simulink model "BD_PAR_AUTO_base_model"  (Simulink 10.3)
settings: Solver=ode1  StartTime=0.0  StopTime=max(cyc_mph(:,1))  FixedStep=1  MaxStep=1  RelTol=1e-3  AbsTol=1e-3
undefined symbols (not defined in the file): acc_dcdc_eff, acc_elec_eff, acc_elec_pwr, acc_mech_eff, acc_mech_pwr, acc_mech_trq, air_cp, amb_tmp, cs_charge_deplete_bool, cs_charge_trq, cs_electric_decel_spd, cs_electric_launch_spd_hi, cs_electric_launch_spd_lo, cs_hi_soc, cs_lo_soc, cs_min_trq_frac, cs_off_trq_frac, cyc_avg_time, cyc_cargo_mass, cyc_elevation_init, cyc_filter_bool, cyc_grade, cyc_mph, enable_sim_stop_distance, enable_sim_stop_max_spd, enable_sim_stop_speed, enable_sim_stop_time, enable_stop, enable_stop_fc, ess_cap_scale, ess_coulombic_eff, ess_init_soc, ess_max_ah_cap, ess_max_volts, ess_min_volts, ess_mod_airflow, ess_mod_cp, ess_mod_init_tmp, ess_module_mass, ess_module_num, ess_on, ess_r_chg, ess_r_dis, ess_res_scale_coef, ess_res_scale_fun, ess_set_tmp, ess_soc, ess_th_calc, ess_th_res_off, ess_th_res_on, ess_tmp, ess_voc, ex_calc, ex_cat_co_frac, ex_cat_ext_cp, ex_cat_ext_emisv, ex_cat_ext_init_tmp, ex_cat_ext_mass, ex_cat_ext_sarea, ex_cat_hc_frac ... (+168)
(part 6 of 15)

== system BD_PAR_AUTO_base_model/motor/ controller <mc> par/N-m drive torque per W input/Block NOTES ==
  note: This block determines the ratio of req'd rotor torque to req'd electrical input power,
      |  which is proportional to efficiency if the motor is providing torque.  This ratio is used
      | to compute actual rotor torque given some input power which may be different from
      | the req'd value.
      |
      | If the denominator, the req'd input power, is zero, this block outputs inf,
      | which is a flag used by the block .../rotor drive torque available (Nm).

== system BD_PAR_AUTO_base_model/motor/ controller <mc> par/effect of inertia (Nm)/Block NOTES ==
  note: Torque required to accelerate the motor's inertia is calculated from the rate of change
      | of mc_spd_out_a.  It is no greater than the product of the maximum motor torque and
      | the fractional contribution of the motor's inertia to the total vehicle inertia.

== system BD_PAR_AUTO_base_model/motor/ controller <mc> par/effect of inertia (Nm)/motor inertia as a function of total vehicle inertia (generous approximation) ==
  gear ratio : Inport
  Product : Product  Inputs=*/  SaturateOnIntegerOverflow=on
  Sum : Sum  Inputs=++|  SaturateOnIntegerOverflow=on
  engine inertia as a fraction of total vehicle inertia  (generous approximation)--denomenator : Fcn  Expr=mc_inertia*u^2
  engine inertia as a fraction of total vehicle inertia  (generous approximation)--numerator : Fcn  Expr=mc_inertia*u^2
  veh mass calc : Subsystem
  Out1 : Outport
  wires:
  Sum/1 -> Product/2
  engine inertia as a fraction of total vehicle inertia  (generous approximation)--denomenator/1 -> Sum/2
  veh mass calc/1(Out1) -> Sum/1
  gear ratio/1 -> engine inertia as a fraction of total vehicle inertia  (generous approximation)--denomenator/1, engine inertia as a fraction of total vehicle inertia  (generous approximation)--numerator/1
  Product/1 -> Out1/1
  engine inertia as a fraction of total vehicle inertia  (generous approximation)--numerator/1 -> Product/1

== system BD_PAR_AUTO_base_model/motor/ controller <mc> par/enforce torque limit/Block NOTES ==
  note: This block enforces the maximum torque production and absorption
      | capability limits of the motor.  It assumes that exactly as much torque
      | can be absorbed as can be produced at a given speed.

== system BD_PAR_AUTO_base_model/motor/ controller <mc> par/mc tmp/Block NOTES ==
  note: This block models the thermal behavior of a motor
      | and controller  with active fluid cooling.
      | The module is modeled as a single lumped thermal mass.
      | The fan is on whenever the battery temp is > the set temp.

== system BD_PAR_AUTO_base_model/motor/ controller <mc> par/mc tmp/mc coolant ==
  Tcl : Inport
  "Qmc " : Inport  Port=2
  Enable : EnablePort  StatesWhenEnabling=reset
  Constant : Constant  Value=mc_tstat
  Product1 : Product  SaturateOnIntegerOverflow=on
  Relational Operator : RelationalOperator  Operator=<=  RndMeth=Nearest  InputSameDT=on
  Qmc_clt : Outport  OutputWhenDisabled=reset  InitialOutput=0
  wires:
  Tcl/1 -> Relational Operator/2
  Constant/1 -> Relational Operator/1
  "Qmc "/1 -> Product1/2
  Product1/1 -> Qmc_clt/1
  Relational Operator/1 -> Product1/1

== system BD_PAR_AUTO_base_model/motor/ controller <mc> par/motor speed estimator/Block NOTES ==
  note: The requested motor speed is replaced by an estimate of the
      | motor's previous speed, for loss and max. torque calculations,
      | whenever the vehicle missed the trace by more than 1 mph
      | on the last time step.

== system BD_PAR_AUTO_base_model/motor/ controller <mc> par/rotor drive torque available (Nm)/Block NOTES ==
  note: This block computes the actual rotor torque given the actual motor input power and
      | the ratio (req'd rotor torque)/(req'd input power).
      |
      | If the above ratio has the value inf, which implies that the req'd input power is zero,
      | then the actual rotor torque is assumed to be zero.  This is not reflective of reality, of course:
      | with zero input power, the rotor torque would be the motor spin-loss torque at the given speed.
      | Because this simplification occurs only when req'd input power is zero, it does not.
      | affect fuel economy or max effort acceleration calculations.

== system BD_PAR_AUTO_base_model/vehicle <veh>/force req'd to accelerate (N)/current veh mass ==
  Constant3 : Constant  Value=veh_mass
  Sum1 : Sum  Inputs=|++  SaturateOnIntegerOverflow=on
  Out1 : Outport
  wires:
  Constant3/1 -> Sum1/1
  [veh_cargo_mass] -> Sum1/2
  Sum1/1 -> Out1/1

== system BD_PAR_AUTO_base_model/vehicle <veh>/force req'd to ascend (N)/current veh mass ==
  Constant3 : Constant  Value=veh_mass
  Sum1 : Sum  Inputs=|++  SaturateOnIntegerOverflow=on
  Out1 : Outport
  wires:
  Constant3/1 -> Sum1/1
  [veh_cargo_mass] -> Sum1/2
  Sum1/1 -> Out1/1

== system BD_PAR_AUTO_base_model/vehicle <veh>/record achieved force outputs/force req'd to accelerate (N)1 ==
  v(m/s) : Inport
  v prev : Inport  Port=2
  Clock : Clock
  Memory : Memory  InitialCondition=-0.1
  Product1 : Product  Inputs=**/  SaturateOnIntegerOverflow=on
  Sum : Sum  Inputs=+-  SaturateOnIntegerOverflow=on
  Sum1 : Sum  Inputs=+-  SaturateOnIntegerOverflow=on
  current veh mass : Subsystem
  (N) : Outport  InitialOutput=0
  wires:
  current veh mass/1(Out1) -> Product1/1
  Clock/1 -> Sum1/1, Memory/1
  Memory/1 -> Sum1/2
  Product1/1 -> (N)/1
  v prev/1 -> Sum/2
  v(m/s)/1 -> Sum/1
  Sum1/1 -> Product1/3
  Sum/1 -> Product1/2

== system BD_PAR_AUTO_base_model/vehicle <veh>/record achieved force outputs/force req'd to ascend (N)1 ==
  average vehicle speed over time step (m/s) : Inport
  Constant : Constant  Value=veh_gravity
  Constant1 : Constant  Value=0
  Product : Product  Inputs=3  SaturateOnIntegerOverflow=on
  Switch : Switch
  Trigonometric Function : Trigonometry  Operator=atan
  Trigonometric Function1 : Trigonometry
  current veh mass : Subsystem
  (N) : Outport  InitialOutput=0
  wires:
  current veh mass/1(Out1) -> Product/3
  average vehicle speed over time step (m/s)/1 -> Switch/2
  Constant1/1 -> Switch/3
  Switch/1 -> (N)/1
  Product/1 -> Switch/1
  Constant/1 -> Product/1
  [grade] -> Trigonometric Function/1
  Trigonometric Function1/1 -> Product/2
  Trigonometric Function/1 -> Trigonometric Function1/1

== system BD_PAR_AUTO_base_model/vehicle <veh>/record achieved force outputs/force req'd to overcome aerodynamic drag (N)1 ==
  average vehicle speed over time step (m/s) : Inport
  Constant : Constant  Value=veh_air_density*veh_CD*veh_FA*0.5
  Product : Product  Inputs=3  SaturateOnIntegerOverflow=on
  D aero(N) : Outport  InitialOutput=0
  wires:
  Product/1 -> D aero(N)/1
  Constant/1 -> Product/3
  average vehicle speed over time step (m/s)/1 -> Product/2, Product/1

== system BD_PAR_AUTO_base_model/vehicle <veh>/record achieved force outputs/rolling resistance force ==
  average vehicle speed over time step (m/s) : Inport
  force req'd to overcome rolling resistance (N) : Subsystem
  Fr (N) : Outport
  wires:
  average vehicle speed over time step (m/s)/1 -> force req'd to overcome rolling resistance (N)/1(average vehicle speed over time step (m/s))
  force req'd to overcome rolling resistance (N)/1(Fr (N)) -> Fr (N)/1

== system BD_PAR_AUTO_base_model/vehicle <veh>/rolling resistance force/force req'd to overcome rolling resistance (N) ==
  average vehicle speed over time step (m/s) : Inport
  Constant : Constant  Value=wh_1st_rrc
  Constant1 : Constant  Value=0
  Constant2 : Constant  Value=veh_gravity
  Gain1 : Gain  Gain=wh_2nd_rrc  SaturateOnIntegerOverflow=on
  Product : Product  Inputs=4  SaturateOnIntegerOverflow=on
  Sum : Sum  SaturateOnIntegerOverflow=on
  Switch : Switch  Threshold=eps
  Trig Fn2 : Trigonometry  Operator=atan
  Trig Fn3 : Trigonometry  Operator=cos
  current veh mass : Subsystem
  Fr (N) : Outport  InitialOutput=0
  wires:
  Constant/1 -> Sum/1
  Gain1/1 -> Sum/2
  Switch/1 -> Fr (N)/1
  average vehicle speed over time step (m/s)/1 -> Gain1/1, Switch/2
  Constant1/1 -> Switch/3
  Sum/1 -> Product/2
  Constant2/1 -> Product/1
  Product/1 -> Switch/1
  Trig Fn3/1 -> Product/3
  current veh mass/1(Out1) -> Product/4
  [grade] -> Trig Fn2/1
  Trig Fn2/1 -> Trig Fn3/1

== system BD_PAR_AUTO_base_model/vehicle <veh>/vehicle speed/vehicle speed (m/s) ==
  vehicle speed at beginning of time step (m/s) : Inport
  "available tractive force and linear speed (N), (m/s)" : Inport  Port=2
  Block NOTES : Subsystem
      mask Display: disp('Block\nNOTES')
  Clock : Clock
  Constant : Constant  Value=0
  Demux : Demux  Outputs=2
  Gain : Gain  Gain=-1  SaturateOnIntegerOverflow=on
  Gain1 : Gain  Gain=2  SaturateOnIntegerOverflow=on
  Memory : Memory  InitialCondition=-.1
  MinMax : MinMax  Inputs=2
  MinMax1 : MinMax  Function=max  Inputs=2
  Mux : Mux  Inputs=3
  Relational Operator : RelationalOperator  RndMeth=Nearest  InputSameDT=on
  Sum5 : Sum  Inputs=-+  SaturateOnIntegerOverflow=on
  Switch : Switch  Threshold=0.5
  Switch1 : Switch  Threshold=1e-9
  Trig Fn4 : Trigonometry  Operator=atan
  a : Constant  Value=0.5*veh_air_density*veh_CD*veh_FA
  b : Subsystem
  c : Subsystem
  current veh mass : Subsystem
  dt : Sum  Inputs=+-  SaturateOnIntegerOverflow=on
  only have rolling resistance if moving : Fcn  Expr=u>0
  solve the quadratic for avg. linear spd : Fcn  Expr=(-u[2]+(u[2]^2-4*u[1]*u[3])^.5)/(2*u[1])
  vehicle speed achievable at end of time step (m/s) : Outport  InitialOutput=0
  wires:
  vehicle speed at beginning of time step (m/s)/1 -> Sum5/1, c/2(v_prev)
  Demux/1 -> c/3(Ftract), Relational Operator/1
  Demux/2 -> MinMax1/2, MinMax/2, only have rolling resistance if moving/1
  c/1(c) -> Mux/3
  "available tractive force and linear speed (N), (m/s)"/1 -> Demux/1
  Constant/1 -> Switch1/3
  Sum5/1 -> Switch1/2, Switch1/1
  only have rolling resistance if moving/1 -> c/5(vehicle moving?), b/3(vehicle moving?)
  Trig Fn4/1 -> c/4(angle of elevation), b/2(angle of elevation)
  dt/1 -> c/1(dt), b/1(dt)
  [grade] -> Trig Fn4/1
  Memory/1 -> dt/2
  Clock/1 -> Memory/1, dt/1
  b/1(b) -> Mux/2
  Switch1/1 -> vehicle speed achievable at end of time step (m/s)/1
  Mux/1 -> solve the quadratic for avg. linear spd/1
  a/1 -> Mux/1
  MinMax/1 -> Switch/1
  MinMax1/1 -> Switch/3
  Gain1/1 -> Sum5/2
  solve the quadratic for avg. linear spd/1 -> MinMax1/1, MinMax/1
  Switch/1 -> Gain1/1
  Gain/1 -> Relational Operator/2
  current veh mass/1(Out1) -> Gain/1
  Relational Operator/1 -> Switch/2

== system BD_PAR_AUTO_base_model/wheel and axle  front/rear <wh>/front force/brake request  controller interface ==
  F_front_brake_req : Outport  InitialOutput=0
  wires:
  [F_front_brake_req] -> F_front_brake_req/1

== system BD_PAR_AUTO_base_model/wheel and axle  front/rear <wh>/loss (Nm)/veh mass calc ==
  Constant : Constant  Value=veh_mass
  Sum : Sum  Inputs=|++  SaturateOnIntegerOverflow=on
  Out1 : Outport
  wires:
  Sum/1 -> Out1/1
  Constant/1 -> Sum/2
  [veh_cargo_mass] -> Sum/1

== system BD_PAR_AUTO_base_model/wheel and axle  front/rear <wh>/rear force/brake request controller interface1 ==
  F_rear_brake_req : Outport  InitialOutput=0
  wires:
  [F_rear_brake_req] -> F_rear_brake_req/1

== system BD_PAR_AUTO_base_model/wheel and axle  front/rear <wh>/tire slip model (m/s)/Block NOTES ==
  note: This block implements the effects of finite tire slip (with respect to the road) on the
      | vehicle speed/wheel speed relationship.  Slip is defined as s=(omega*r - v) / v.  The
      | one-to-one mapping of slip to normalized tractive force, F_tract/W_front_axle, up to
      | the maximum, is stored in the variables "wh_slip" and "wh_slip_force_coeff."  The
      | slip calculation here is overridden if the actual axle speed and the requested axle
      | speed are the same, indicating that no drivetrain speed limits were encountered.

== system BD_PAR_AUTO_base_model/wheel and axle  front/rear <wh>/tire slip model (m/s)/front axle ==
  In1 : Inport
  In2 : Inport  Port=2
  Abs : Abs
  Constant3 : Constant  Value=0
  F/W : Product  Inputs=*/  SaturateOnIntegerOverflow=on
  Product : Product  SaturateOnIntegerOverflow=on
  Relational Operator : RelationalOperator  Operator=~=  RndMeth=Nearest  InputSameDT=on
  Saturation : Saturate  UpperLimit=max(wh_slip_force_coeff)  LowerLimit=min(wh_slip_force_coeff)
  Sign : Signum
  Switch : Switch
  s=s(F/W) : Lookup  InputValues=wh_slip_force_coeff  Table=wh_slip
  Out1 : Outport
  wires:
  Product/1 -> Out1/1
  In1/1 -> F/W/2
  In2/1 -> Sign/1, Abs/1
  s=s(F/W)/1 -> Product/1
  Sign/1 -> Product/2
  F/W/1 -> Switch/1
  Switch/1 -> Saturation/1
  Saturation/1 -> s=s(F/W)/1
  Abs/1 -> Relational Operator/1, F/W/1
  Relational Operator/1 -> Switch/2
  Constant3/1 -> Relational Operator/2, Switch/3

== system BD_PAR_AUTO_base_model/wheel and axle  front/rear <wh>/tire slip model (m/s)/rear axle ==
  In1 : Inport
  In2 : Inport  Port=2
  Abs : Abs
  Constant3 : Constant  Value=0
  F/W : Product  Inputs=*/  SaturateOnIntegerOverflow=on
  Product : Product  SaturateOnIntegerOverflow=on
  Relational Operator : RelationalOperator  Operator=~=  RndMeth=Nearest  InputSameDT=on
  Saturation : Saturate  UpperLimit=max(wh_slip_force_coeff)  LowerLimit=min(wh_slip_force_coeff)
  Sign : Signum
  Switch : Switch
  s=s(F/W) : Lookup  InputValues=wh_slip_force_coeff  Table=wh_slip
  Out1 : Outport
  wires:
  Product/1 -> Out1/1
  In1/1 -> F/W/2
  In2/1 -> Sign/1, Abs/1
  s=s(F/W)/1 -> Product/1
  Sign/1 -> Product/2
  F/W/1 -> Switch/1
  Switch/1 -> Saturation/1
  Saturation/1 -> s=s(F/W)/1
  Abs/1 -> Relational Operator/1, F/W/1
  Relational Operator/1 -> Switch/2
  Constant3/1 -> Relational Operator/2, Switch/3

== system BD_PAR_AUTO_base_model/wheel and axle  front/rear <wh>/tire slip model (rad/s)/front slip ==
  In1 : Inport
  In2 : Inport  Port=2
  Abs : Abs
  F/W : Product  Inputs=*/  SaturateOnIntegerOverflow=on
  Product : Product  SaturateOnIntegerOverflow=on
  Saturation : Saturate  UpperLimit=max(wh_slip_force_coeff)  LowerLimit=min(wh_slip_force_coeff)
  Sign : Signum
  s=s(F/W) : Lookup  InputValues=wh_slip_force_coeff  Table=wh_slip
  Out1 : Outport
  wires:
  Product/1 -> Out1/1
  In1/1 -> F/W/2
  s=s(F/W)/1 -> Product/1
  In2/1 -> Sign/1, Abs/1
  Sign/1 -> Product/2
  Abs/1 -> F/W/1
  F/W/1 -> Saturation/1
  Saturation/1 -> s=s(F/W)/1

== system BD_PAR_AUTO_base_model/wheel and axle  front/rear <wh>/tire slip model (rad/s)/rear slip ==
  In1 : Inport
  In2 : Inport  Port=2
  Abs : Abs
  F/W : Product  Inputs=*/  SaturateOnIntegerOverflow=on
  Product : Product  SaturateOnIntegerOverflow=on
  Saturation : Saturate  UpperLimit=max(wh_slip_force_coeff)  LowerLimit=min(wh_slip_force_coeff)
  Sign : Signum
  s=s(F/W) : Lookup  InputValues=wh_slip_force_coeff  Table=wh_slip
  Out1 : Outport
  wires:
  Product/1 -> Out1/1
  In1/1 -> F/W/2
  s=s(F/W)/1 -> Product/1
  In2/1 -> Sign/1, Abs/1
  Sign/1 -> Product/2
  Abs/1 -> F/W/1
  F/W/1 -> Saturation/1
  Saturation/1 -> s=s(F/W)/1

== system BD_PAR_AUTO_base_model/<vc> par auto/config traction control/traction control 2 axle/Block NOTES ==
  note: Requested speed and force are limited by the
      | tractive characteristics of the tires in this block.

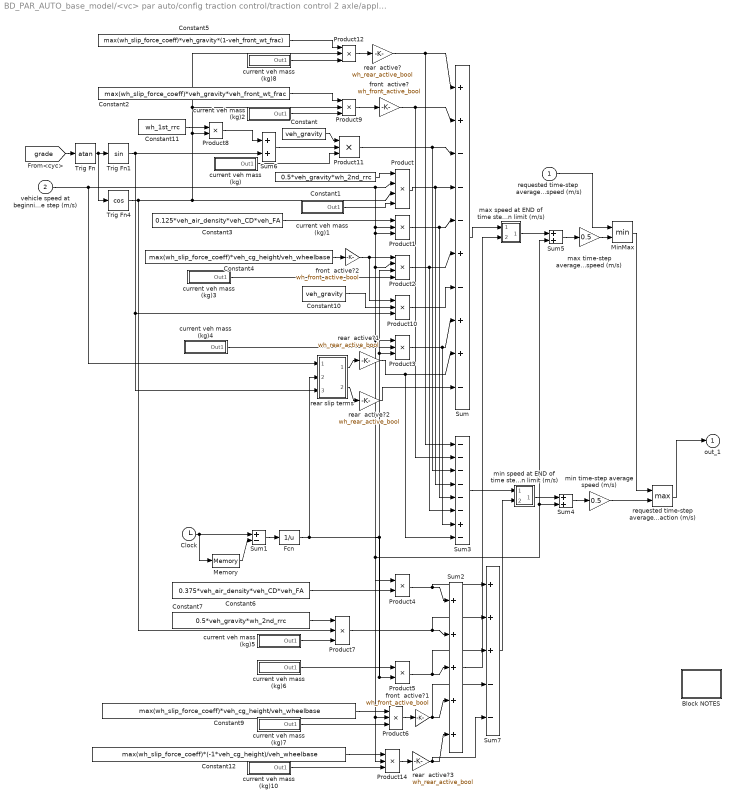
== system BD_PAR_AUTO_base_model/<vc> par auto/config traction control/traction control 2 axle/apply tire traction limit to req'd speed (m/s) ==
  "requested time-step  average vehicle speed (m/s) " : Inport
  vehicle speed at beginning of time step (m/s) : Inport  Port=2
  Block NOTES : Subsystem
      mask Display: disp('Block\nNOTES')
  Clock : Clock
  Constant : Constant  Value=veh_gravity
  Constant1 : Constant  Value=0.5*veh_gravity*wh_2nd_rrc
  Constant10 : Constant  Value=veh_gravity
  Constant11 : Constant  Value=wh_1st_rrc
  Constant12 : Constant  Value=max(wh_slip_force_coeff)*(-1*veh_cg_height)/veh_wheelbase
  Constant2 : Constant  Value=max(wh_slip_force_coeff)*veh_gravity*veh_front_wt_frac
  Constant3 : Constant  Value=0.125*veh_air_density*veh_CD*veh_FA
  Constant4 : Constant  Value=max(wh_slip_force_coeff)*veh_cg_height/veh_wheelbase
  Constant5 : Constant  Value=max(wh_slip_force_coeff)*veh_gravity*(1-veh_front_wt_frac)
  Constant6 : Constant  Value=0.375*veh_air_density*veh_CD*veh_FA
  Constant7 : Constant  Value=0.5*veh_gravity*wh_2nd_rrc
  Constant9 : Constant  Value=max(wh_slip_force_coeff)*veh_cg_height/veh_wheelbase
  Fcn : Fcn  Expr=1/u
  Memory : Memory  InitialCondition=-0.1
  MinMax : MinMax  Inputs=2  InputSameDT=on  SaturateOnIntegerOverflow=on
  Product : Product  Inputs=4  InputSameDT=on  RndMeth=Zero  SaturateOnIntegerOverflow=on  OutDataTypeStr=Inherit: Same as first input
  Product{1,3,6..7,9..12,14} (9 alike) : Product  Inputs=3  InputSameDT=on  RndMeth=Zero  SaturateOnIntegerOverflow=on  OutDataTypeStr=Inherit: Same as first input
  Product2 : Product  Inputs=4  InputSameDT=on  RndMeth=Zero  SaturateOnIntegerOverflow=on  OutDataTypeStr=Inherit: Same as first input
  Product4 : Product  InputSameDT=on  RndMeth=Zero  SaturateOnIntegerOverflow=on  OutDataTypeStr=Inherit: Same as first input
  Product5 : Product  InputSameDT=on  RndMeth=Zero  SaturateOnIntegerOverflow=on  OutDataTypeStr=Inherit: Same as first input
  Product8 : Product  InputSameDT=on  RndMeth=Zero  SaturateOnIntegerOverflow=on  OutDataTypeStr=Inherit: Same as first input
  Sum : Sum  Inputs=++---+-++-  InputSameDT=on  SaturateOnIntegerOverflow=on  OutDataTypeStr=Inherit: Same as first input
  Sum1 : Sum  Inputs=+-  InputSameDT=on  SaturateOnIntegerOverflow=on  OutDataTypeStr=Inherit: Same as first input
  Sum2 : Sum  Inputs=+++++  InputSameDT=on  SaturateOnIntegerOverflow=on  OutDataTypeStr=Inherit: Same as first input
  Sum3 : Sum  Inputs=------+-  InputSameDT=on  SaturateOnIntegerOverflow=on  OutDataTypeStr=Inherit: Same as first input
  Sum4 : Sum  InputSameDT=on  SaturateOnIntegerOverflow=on  OutDataTypeStr=Inherit: Same as first input
  Sum5 : Sum  InputSameDT=on  SaturateOnIntegerOverflow=on  OutDataTypeStr=Inherit: Same as first input
  Sum6 : Sum  InputSameDT=on  SaturateOnIntegerOverflow=on  OutDataTypeStr=Inherit: Same as first input
  Sum7 : Sum  Inputs=+++--  InputSameDT=on  SaturateOnIntegerOverflow=on  OutDataTypeStr=Inherit: Same as first input
  Trig Fn4 : Trigonometry  Operator=cos
  Trig Fn : Trigonometry  Operator=atan
  Trig Fn1 : Trigonometry
  current veh mass (kg) : Subsystem
  current veh mass (kg)1 : Subsystem
  current veh mass (kg)10 : Subsystem
  current veh mass (kg)2 : Subsystem
  current veh mass (kg)3 : Subsystem
  current veh mass (kg)4 : Subsystem
  current veh mass (kg)5 : Subsystem
  current veh mass (kg)6 : Subsystem
  current veh mass (kg)7 : Subsystem
  current veh mass (kg)8 : Subsystem
  front  active? : Gain  Gain=wh_front_active_bool  SaturateOnIntegerOverflow=on  OutDataTypeStr=Inherit: Same as input  ParamDataTypeStr=Inherit: Same as input
  front  active?1 : Gain  Gain=wh_front_active_bool  SaturateOnIntegerOverflow=on  OutDataTypeStr=Inherit: Same as input  ParamDataTypeStr=Inherit: Same as input
  front  active?2 : Gain  Gain=wh_front_active_bool  SaturateOnIntegerOverflow=on  OutDataTypeStr=Inherit: Same as input  ParamDataTypeStr=Inherit: Same as input
  max speed at END of time step given tire traction limit (m/s) : Subsystem
      mask Display: disp('/')
  max time-step average speed (m/s) : Gain  Gain=0.5  SaturateOnIntegerOverflow=on  OutDataTypeStr=Inherit: Same as input  ParamDataTypeStr=Inherit: Same as input
  min speed at END of time step given tire traction limit (m/s) : Subsystem
      mask Display: disp('/')
  min time-step average speed (m/s) : Gain  Gain=0.5  SaturateOnIntegerOverflow=on  OutDataTypeStr=Inherit: Same as input  ParamDataTypeStr=Inherit: Same as input
  rear  active?{,1..3} (4 alike) : Gain  Gain=wh_rear_active_bool  SaturateOnIntegerOverflow=on  OutDataTypeStr=Inherit: Same as input  ParamDataTypeStr=Inherit: Same as input
  rear slip terms : Subsystem
  requested time-step average speed limited by tire traction (m/s) : MinMax  Function=max  Inputs=2  InputSameDT=on  SaturateOnIntegerOverflow=on
  out_1 : Outport  InitialOutput=0
  wires:
  front  active?2/1 -> Product10/1, Product2/1
  front  active?1/1 -> Sum2/4, Sum7/4
  front  active?/1 -> Sum3/2, Sum/2
  rear  active?3/1 -> Sum2/5, Sum7/5
  rear  active?2/1 -> Sum/10
  rear  active?1/1 -> Sum3/8, Sum/9
  current veh mass (kg)10/1(Out1) -> Product14/3
  Constant12/1 -> Product14/1
  Product14/1 -> rear  active?3/1
  rear slip terms/2(Out2) -> rear  active?2/1
  rear slip terms/1(Out1) -> rear  active?1/1
  rear  active?/1 -> Sum3/1, Sum/1
  current veh mass (kg)8/1(Out1) -> Product12/3
  Constant5/1 -> Product12/1
  Product12/1 -> rear  active?/1
  current veh mass (kg)7/1(Out1) -> Product6/3
  current veh mass (kg)5/1(Out1) -> Product7/3
  current veh mass (kg)3/1(Out1) -> Product2/4
  current veh mass (kg)2/1(Out1) -> Product9/3
  current veh mass (kg)1/1(Out1) -> Product/4
  current veh mass (kg)/1(Out1) -> Product11/3
  Constant/1 -> Product11/1
  Product11/1 -> Sum3/3, Sum/3
  Sum6/1 -> Product11/2
  Trig Fn1/1 -> rear slip terms/3(sin(theta)), Product10/3, Sum6/2
  Constant10/1 -> Product10/2
  Constant4/1 -> front  active?2/1
  Product10/1 -> Sum/7
  Product3/1 -> Sum3/7, Sum/8
  current veh mass (kg)4/1(Out1) -> Product3/2
  max time-step average speed (m/s)/1 -> MinMax/2
  "requested time-step  average vehicle speed (m/s) "/1 -> MinMax/1
  Sum5/1 -> max time-step average speed (m/s)/1
  Constant2/1 -> Product9/1
  Constant11/1 -> Product8/1
  Product8/1 -> Sum6/1
  Trig Fn4/1 -> Product12/2, Product9/2, Product8/2, Product/3, Product7/2
  Clock/1 -> Memory/1, Sum1/1
  Sum1/1 -> Fcn/1
  Memory/1 -> Sum1/2
  current veh mass (kg)6/1(Out1) -> Product5/1
  Sum2/1 -> max speed at END of time step given tire traction limit (m/s)/2(in_2)
  min time-step average speed (m/s)/1 -> requested time-step average speed limited by tire traction (m/s)/2
  requested time-step average speed limited by tire traction (m/s)/1 -> out_1/1
  Sum4/1 -> min time-step average speed (m/s)/1
  min speed at END of time step given tire traction limit (m/s)/1(out_1) -> Sum4/1
  MinMax/1 -> requested time-step average speed limited by tire traction (m/s)/1
  Sum3/1 -> min speed at END of time step given tire traction limit (m/s)/1(in_1)
  Sum7/1 -> min speed at END of time step given tire traction limit (m/s)/2(in_2)
  Constant7/1 -> Product7/1
  Constant9/1 -> Product6/1
  Constant6/1 -> Product4/2
  Product4/1 -> Sum2/1, Sum7/1
  Product7/1 -> Sum2/2, Sum7/2
  Product5/1 -> Sum2/3, Sum7/3
  Product6/1 -> front  active?1/1
  Trig Fn/1 -> Trig Fn4/1, Trig Fn1/1
  vehicle speed at beginning of time step (m/s)/1 -> rear slip terms/1(initial speed), Sum5/2, Sum4/2, Product4/1, Product3/1, Product2/2, Product1/3, Product1/2, Product/2
  [grade] -> Trig Fn/1
  max speed at END of time step given tire traction limit (m/s)/1(out_1) -> Sum5/1
  Product2/1 -> Sum3/6, Sum/6
  Product9/1 -> front  active?/1
  Product/1 -> Sum3/4, Sum/4
  Product1/1 -> Sum3/5, Sum/5
  Sum/1 -> max speed at END of time step given tire traction limit (m/s)/1(in_1)
  Fcn/1 -> rear slip terms/2(1/dt), Product14/2, Product6/2, Product5/2, Product3/3, Product2/3
  Constant3/1 -> Product1/1
  Constant1/1 -> Product/1

== system BD_PAR_AUTO_base_model/<vc> par auto/config traction control/traction control 2 axle/enforce max.  front axle tractive force  due to slip (N) ==
  tractive force req'd at tire/road interface (N) : Inport
  requested time-step average vehicle speed (m/s) : Inport  Port=2
  speed at beginning of time step (m/s) : Inport  Port=3
  " " : MinMax  Inputs=2  InputSameDT=on  SaturateOnIntegerOverflow=on
  Block NOTES : Subsystem
      mask Display: disp('Block\nNOTES')
  Constant2 : Constant  Value=max(wh_slip_force_coeff)
  Gain : Gain  Gain=-1  SaturateOnIntegerOverflow=on  OutDataTypeStr=Inherit: Same as input  ParamDataTypeStr=Inherit: Same as input
  Product1 : Product  InputSameDT=on  RndMeth=Zero  SaturateOnIntegerOverflow=on  OutDataTypeStr=Inherit: Same as first input
  Product2 : Product  InputSameDT=on  RndMeth=Zero  SaturateOnIntegerOverflow=on  OutDataTypeStr=Inherit: Same as first input
  Product3 : Product  Inputs=*/  InputSameDT=on  RndMeth=Zero  SaturateOnIntegerOverflow=on  OutDataTypeStr=Inherit: Same as first input
  Product4 : Product  Inputs=*/  InputSameDT=on  RndMeth=Zero  SaturateOnIntegerOverflow=on  OutDataTypeStr=Inherit: Same as first input
  Sum1 : Sum  InputSameDT=on  SaturateOnIntegerOverflow=on  OutDataTypeStr=Inherit: Same as first input
  Sum2 : Sum  InputSameDT=on  SaturateOnIntegerOverflow=on  OutDataTypeStr=Inherit: Same as first input
  front : Subsystem
  front  active? : Gain  Gain=wh_front_active_bool  SaturateOnIntegerOverflow=on  OutDataTypeStr=Inherit: Same as input  ParamDataTypeStr=Inherit: Same as input
  front traction ratio : ToWorkspace  VariableName=front_traction_ratio_orig
  rear : Subsystem
  rear  active? : Gain  Gain=wh_rear_active_bool  SaturateOnIntegerOverflow=on  OutDataTypeStr=Inherit: Same as input  ParamDataTypeStr=Inherit: Same as input
  tractive force request limited by slip-threshhold force (N)1 : MinMax  Function=max  Inputs=2  InputSameDT=on  SaturateOnIntegerOverflow=on
  slip-limited force (N) : Outport  InitialOutput=0
  weight on front axle (N) : Outport  Port=2  InitialOutput=0
  weight on rear axle (N) : Outport  Port=3  InitialOutput=0
  front/total traction ratio : Outport  Port=4  InitialOutput=0
  wires:
  Product4/1 -> front traction ratio/1
  Sum2/1 -> Product4/2
  rear  active?/1 -> Sum1/2
  front  active?/1 -> Product3/1, Sum1/1
  Product3/1 -> front/total traction ratio/1
  Product2/1 -> Product4/1, Sum2/1, front  active?/1
  Product1/1 -> Sum2/2, rear  active?/1
  Sum1/1 -> Product3/2, Gain/1, " "/1
  rear/1(Out1) -> Product1/1, weight on rear axle (N)/1
  tractive force request limited by slip-threshhold force (N)1/1 -> slip-limited force (N)/1
  " "/1 -> tractive force request limited by slip-threshhold force (N)1/1
  tractive force req'd at tire/road interface (N)/1 -> " "/2
  Constant2/1 -> Product1/2, Product2/2
  Gain/1 -> tractive force request limited by slip-threshhold force (N)1/2
  speed at beginning of time step (m/s)/1 -> rear/2(In2), front/2(In2)
  requested time-step average vehicle speed (m/s)/1 -> rear/1(In1), front/1(In1)
  front/1(Out1) -> weight on front axle (N)/1, Product2/1

== system BD_PAR_AUTO_base_model/<vc> par auto/front and rear brake controller (achievable)/braking force supplied by front friction brakes (N)/Block NOTES ==
  note: If additional braking force is required to meet the specified deceleration, input #1 will be negative.
      | The fraction of the additional req'd braking force made up by the front-axle friction brakes is given by:
  note: [front_axle_friction_brake_fraction(vehicle speed)]
      | ------------------------------------------------------------------------------
      | [front_axle_friction_brake_fraction(vehicle speed) + rear_axle_friction_brake_fraction(vehicle speed)]
  note: where the denominator can also be expressed as [1 - front_axle_drivetrain_brake_fraction(vehicle speed)].
  note: If all braking was intended to be done by the drivetrain, the front friction brakes will do 60% of the braking.
  note: The variable "wh_max_front_fric_brake_force_N" must be assigned a positive value.

== system BD_PAR_AUTO_base_model/<vc> par auto/gearbox control for use w/ AT/Speed Dependent Shifting/shifting ==
  gear number : Inport
  Constant : Constant  Value=gb_shift_delay-1e-6
  Relational Operator : RelationalOperator  Operator=<  RndMeth=Nearest  InputSameDT=on
  time since last shift : Subsystem
      mask Display: disp('time since\nlast shift')
  out_1 : Outport  InitialOutput=0
  wires:
  time since last shift/1(out_1) -> Relational Operator/1
  Constant/1 -> Relational Operator/2
  gear number/1 -> time since last shift/1(in_1)
  Relational Operator/1 -> out_1/1

== system BD_PAR_AUTO_base_model/<vc> par auto/gearbox control for use w/ AT/Speed Dependent Shifting/shifting1 ==
  gear number : Inport
  Constant : Constant  Value=gb_shift_delay-1e-6
  Relational Operator : RelationalOperator  Operator=<  RndMeth=Nearest  InputSameDT=on
  time since last shift : Subsystem
      mask Display: disp('time since\nlast shift')
  out_1 : Outport  InitialOutput=0
  wires:
  time since last shift/1(out_1) -> Relational Operator/1
  Constant/1 -> Relational Operator/2
  gear number/1 -> time since last shift/1(in_1)
  Relational Operator/1 -> out_1/1

== system BD_PAR_AUTO_base_model/<vc> par auto/gearbox control for use w/ AT/downshift  command/load fraction ==
  In1 : Inport
  S-Function : S-Function  FunctionName=sfun_gearbox  Parameters=load, spd  SFunctionDeploymentMode=off  EnableBusSupport=off
  Out1 : Outport  InitialOutput=0
  wires:
  In1/1 -> S-Function/1
  S-Function/1 -> Out1/1

== system BD_PAR_AUTO_base_model/<vc> par auto/gearbox control for use w/ AT/downshift  command1/load fraction ==
  In1 : Inport
  S-Function : S-Function  FunctionName=sfun_gearbox  Parameters=load, spd  SFunctionDeploymentMode=off  EnableBusSupport=off
  Out1 : Outport  InitialOutput=0
  wires:
  S-Function/1 -> Out1/1
  In1/1 -> S-Function/1

== system BD_PAR_AUTO_base_model/<vc> par auto/gearbox control for use w/ AT/est. engine trq and spd/Block NOTES ==
  note: Estimate engine torque and speed associated with the previous gear, assuming that
      | the gearbox efficiency is constant.

== system BD_PAR_AUTO_base_model/<vc> par auto/gearbox control for use w/ AT/est. engine trq and spd/K_adv ==
  "Req'd output trq and spd (Nm), (rad/s)" : Inport
  K_adv=wout/(Tout)^0.5 : Fcn  Expr=u[2]/u[1]^0.5
  Saturation : Saturate  UpperLimit=max(htc_k_adv)  LowerLimit=min(htc_k_adv)
  Saturation2 : Saturate  UpperLimit=inf  LowerLimit=eps
  K_adv : Outport
  wires:
  Saturation/1 -> K_adv/1
  K_adv=wout/(Tout)^0.5/1 -> Saturation/1
  Saturation2/1 -> K_adv=wout/(Tout)^0.5/1
  "Req'd output trq and spd (Nm), (rad/s)"/1 -> Saturation2/1

== system BD_PAR_AUTO_base_model/<vc> par auto/gearbox control for use w/ AT/est. engine trq and spd assuming lockup/Block NOTES ==
  note: Estimate engine torque and speed associated with the current gear, assuming that
      | the gearbox efficiency is constant.

== system BD_PAR_AUTO_base_model/<vc> par auto/gearbox control for use w/ AT/shifting1/time since last shift ==
  in_1 : Inport
  just shifted : Subsystem
      mask Display: disp('just\nshifted')
  timer : Subsystem
      mask Display: disp('timer')
  out_1 : Outport  InitialOutput=0
  wires:
  timer/1(time) -> out_1/1
  just shifted/1(out_1) -> timer/1(trigger)
  in_1/1 -> just shifted/1(in_1)

== system BD_PAR_AUTO_base_model/<vc> par auto/gearbox control for use w/ AT/upshift  command/load fraction ==
  In1 : Inport
  S-Function : S-Function  FunctionName=sfun_gearbox  Parameters=load, spd  SFunctionDeploymentMode=off  EnableBusSupport=off
  Out1 : Outport  InitialOutput=0
  wires:
  In1/1 -> S-Function/1
  S-Function/1 -> Out1/1

== system BD_PAR_AUTO_base_model/<vc> par auto/parallel clutch control/gearbox speed estimator/Block NOTES ==
  note: The requested engine speed is replaced by an estimate of the
      | engine's previous speed whenever the vehicle missed the trace
      |  by more than 1 mph on the last time step.

== system BD_PAR_AUTO_base_model/<vc> par auto/parallel clutch control/gearbox speed estimator/dt ==
  Clock : Clock
  Memory1 : Memory  InitialCondition=-1
  Sum4 : Sum  Inputs=+-  InputSameDT=on  SaturateOnIntegerOverflow=on  OutDataTypeStr=Inherit: Same as first input
  Out1 : Outport  InitialOutput=0
  wires:
  Sum4/1 -> Out1/1
  Memory1/1 -> Sum4/2
  Clock/1 -> Memory1/1, Sum4/1

== system BD_PAR_AUTO_base_model/<vc> par auto/sim stop subsystem/stop sim max spd/Block NOTES ==
  note: When enabled, stop the simulation when the current speed is greater
      | than zero and is less than or equal to the speed at gb_shift_delay*5+1
      | seconds ago (i.e. vehicle has reached a constant max speed). Only used
      | during acceleration test.

== system BD_PAR_AUTO_base_model/electric acc loads <acc>/Electrical Accessory Loads v2 <acc>/Accessory SDO/electrical power logging ==
  In1 : Inport
  Gain : Gain  Gain=acc_elec_eff  SaturateOnIntegerOverflow=on  OutDataTypeStr=Inherit: Same as input  ParamDataTypeStr=Inherit: Same as input
  To Workspace6 : ToWorkspace  VariableName=acc_elec_pwr_in_a  SampleTime=-1
  To Workspace8 : ToWorkspace  VariableName=acc_elec_pwr_out_a  SampleTime=-1
  wires:
  Gain/1 -> To Workspace8/1
  In1/1 -> Gain/1, To Workspace6/1

== system BD_PAR_AUTO_base_model/electric acc loads <acc>/Electrical Accessory Loads v2 <acc>/backward model/electrical accessories (W) ==
  Electrical Accessories: Time Variable : Subsystem
      mask Display: image(imread('bdi_acc_elec_cs.bmp'))
  P_elec_acc : Outport
  wires:
  Electrical Accessories: Time Variable/1(P_elec_acc) -> P_elec_acc/1

== system BD_PAR_AUTO_base_model/energy storage <ess>/ess config/energy storage <ess>/Block NOTES ==
  note: This block models the energy storage system as an SOC-dependent voltage
      | in series with an SOC- and current direction-dependent internal resistance.
      | SOC is computed assuming that A-h capacity is constant, but limited
      | such that a minimum voltage is never exceeded (replacing the
      | previous Peukert relationship which underpredicted battery capacity).
      |
      | Discharge power is limited here so as not to bring the bus (battery pack) voltage below
      | the minimum controller voltage or the minimum battery voltage and so as to allow
      | the solution of the quadratic eq'n for discharge current.
      |
      | Charge current is limited to ensure the voltage does not exceed a maximum
      | voltage
      |
      | Positive current is discharge current in the convention used here.
      | Power loss is computed as I*R+losses due to Coulombic (in)efficiency.
      |
      | Thermal modeling of the battery performance is modeled in the
      | OCV, Rint, and capacity.

== system BD_PAR_AUTO_base_model/energy storage <ess>/ess config/energy storage <ess>/SOC algorithm ==
  note: SOC=(Max Ah capacity-Ah used)/Max Ah capacity
  (A) : Inport
  tmp (C) : Inport  Port=2
  (sec->hrs) : Gain  Gain=1/3600  SaturateOnIntegerOverflow=on  OutDataTypeStr=Inherit: Same as input  ParamDataTypeStr=Inherit: Same as input
  0 <= SOC <= 1 : Saturate  UpperLimit=1  LowerLimit=0
  A-h remaining : Sum  Inputs=-+  InputSameDT=on  SaturateOnIntegerOverflow=on  OutDataTypeStr=Inherit: Same as first input
  Ah used : Integrator  InitialConditionSource=external  InitialCondition=(1-ess_init_soc)*ess_max_ah_cap
  Fcn : Fcn  Expr=1/u
  Fcn1 : Fcn  Expr=(1-ess_init_soc)*u
  SOC : Product  InputSameDT=on  RndMeth=Zero  SaturateOnIntegerOverflow=on  OutDataTypeStr=Inherit: Same as first input
  Switch : Switch
  adjusted A : Product  InputSameDT=on  RndMeth=Zero  SaturateOnIntegerOverflow=on  OutDataTypeStr=Inherit: Same as first input
  coul eff : Lookup  InputValues=ess_tmp  Table=ess_coulombic_eff
  max cap : Lookup  InputValues=ess_tmp  Table=ess_max_ah_cap*ess_cap_scale
  SOC1 : Outport  InitialOutput=0
  wires:
  (A)/1 -> Switch/2, Switch/1, adjusted A/1
  Switch/1 -> (sec->hrs)/1
  (sec->hrs)/1 -> Ah used/1
  Ah used/1 -> A-h remaining/1
  Fcn/1 -> SOC/2
  SOC/1 -> 0 <= SOC <= 1/1
  A-h remaining/1 -> SOC/1
  0 <= SOC <= 1/1 -> SOC1/1
  tmp (C)/1 -> max cap/1, coul eff/1
  coul eff/1 -> adjusted A/2
  adjusted A/1 -> Switch/3
  max cap/1 -> A-h remaining/2, Fcn/1, Fcn1/1
  Fcn1/1 -> Ah used/2

== system BD_PAR_AUTO_base_model/energy storage <ess>/ess config/energy storage <ess>/compute current ==
  Voc : Inport
  Rint : Inport  Port=2
  limited output power (W) : Inport  Port=3
  Ibty=(Voc-(Voc^2-4RPbty)^.5)        ----------------------------- (2*R) : Fcn  Expr=(u[2]-(u[2]^2-4*u[1]*u[3])^.5)/(2*u[3])
  Logical Operator1 : Logic  Operator=NOT  Inputs=1
  Mux3 : Mux  Inputs=3
  Mux4 : Mux  Inputs=3
  Mux5 : Mux  Inputs=3
  To Workspace9 : ToWorkspace  VariableName=ess_current  SampleTime=-1
  Voc-I*R : Fcn  Expr=u[2]-u[1]*u[3]
  ess max voltage*#batts : Constant  Value=ess_max_volts*ess_module_num
  iabs min=(Voc-Vmax)/R : Fcn  Expr=(u(1)-u(2))/u(3)
  limit current based on  max voltage during charge : Switch  Threshold=eps
  min charge current not exceeded : RelationalOperator  Operator=>  RndMeth=Nearest  InputSameDT=on
  I_ : Outport  InitialOutput=0
  V_ : Outport  Port=2  InitialOutput=0
  tag scope: ess_maxV_limited=global
  wires:
  limited output power (W)/1 -> Mux4/1
  Voc/1 -> Mux4/2, Mux3/2, Mux5/1
  Rint/1 -> Mux4/3, Mux3/3, Mux5/3
  Ibty=(Voc-(Voc^2-4RPbty)^.5)        ----------------------------- (2*R)/1 -> min charge current not exceeded/1, limit current based on  max voltage during charge/1
  iabs min=(Voc-Vmax)/R/1 -> min charge current not exceeded/2, limit current based on  max voltage during charge/3
  limit current based on  max voltage during charge/1 -> I_/1, To Workspace9/1, Mux3/1
  min charge current not exceeded/1 -> limit current based on  max voltage during charge/2, Logical Operator1/1
  Mux3/1 -> Voc-I*R/1
  Voc-I*R/1 -> V_/1
  Mux4/1 -> Ibty=(Voc-(Voc^2-4RPbty)^.5)        ----------------------------- (2*R)/1
  Mux5/1 -> iabs min=(Voc-Vmax)/R/1
  ess max voltage*#batts/1 -> Mux5/2
  Logical Operator1/1 -> [ess_maxV_limited]

== system BD_PAR_AUTO_base_model/energy storage <ess>/ess config/energy storage <ess>/documentation9 ==

== system BD_PAR_AUTO_base_model/energy storage <ess>/ess config/energy storage <ess>/ess tmp ==
  Qess_gen : Inport
  Enable : EnablePort  StatesWhenEnabling=reset
  #of mods : Gain  Gain=ess_module_num  SaturateOnIntegerOverflow=on  OutDataTypeStr=Inherit: Same as input  ParamDataTypeStr=Inherit: Same as input
  1/#of mods : Gain  Gain=1/ess_module_num  SaturateOnIntegerOverflow=on  OutDataTypeStr=Inherit: Same as input  ParamDataTypeStr=Inherit: Same as input
  1/mcp : Gain  Gain=1/(ess_module_mass*ess_mod_cp)  SaturateOnIntegerOverflow=on  OutDataTypeStr=Inherit: Same as input  ParamDataTypeStr=Inherit: Same as input
  Block NOTES : Subsystem
      mask Display: disp('Block\nNOTES')
  Memory : Memory  InitialCondition=cyc_mph(1,2)*.447
  Memory1 : Memory  InitialCondition=cyc_mph(1,2)*.447
  Mux20 : Mux  Inputs=3
  Qc : Sum  InputSameDT=on  SaturateOnIntegerOverflow=on  OutDataTypeStr=Inherit: Same as first input
  Qess_case : Fcn  Expr=(u(2) - u(1))/u(3)
  Saturation3 : Saturate  UpperLimit=1  LowerLimit=0
  Tair,ave : Subsystem  TreatAsAtomicUnit=on
  Tess2 : Integrator  InitialCondition=ess_mod_init_tmp
  thermostat : Fcn  Expr=u(1) - ess_set_tmp
  Tess : Outport  InitialOutput=0
  Tair : Outport  Port=2
  Qair : Outport  Port=3  OutputWhenDisabled=reset  InitialOutput=0
  wires:
  Tair,ave/1(Tair_ave) -> Mux20/2
  Tair,ave/3(Tair) -> Tair/1
  Qc/1 -> 1/mcp/1
  Qess_case/1 -> Qc/1, Memory/1, #of mods/1
  1/mcp/1 -> Tess2/1
  Tess2/1 -> Tess/1, Mux20/1, thermostat/1
  Qess_gen/1 -> 1/#of mods/1
  1/#of mods/1 -> Qc/2
  thermostat/1 -> Saturation3/1
  Saturation3/1 -> Memory1/1
  Memory1/1 -> Tair,ave/Enable
  Memory/1 -> Tair,ave/2(Qess_case1), Tair,ave/1(Qess_case)
  #of mods/1 -> Qair/1
  Mux20/1 -> Qess_case/1
  Tair,ave/2(Th Res) -> Mux20/3

== system BD_PAR_AUTO_base_model/energy storage <ess>/ess config/energy storage <ess>/limit power ==
  SOC : Inport
  Pbty : Inport  Port=2
  Voc : Inport  Port=3
  Rint : Inport  Port=4
  Constant1 : Constant  Value=eps
  Constant{2..4,6} (4 alike) : Constant  Value=0
  Constant5 : Constant  Value=.999
  Gain : Gain  Gain=0.5  SaturateOnIntegerOverflow=on  OutDataTypeStr=Inherit: Same as input  ParamDataTypeStr=Inherit: Same as input
  Limits : Subsystem
  Logical Operator : Logic  Operator=OR
  Logical Operator1 : Logic
  Mux : Mux  Inputs=3
  Relational Operator : RelationalOperator  Operator=>  RndMeth=Nearest  InputSameDT=on
  Relational Operator3 : RelationalOperator  Operator=<  RndMeth=Nearest  InputSameDT=on
  SOC>=.999 : RelationalOperator  RndMeth=Nearest  InputSameDT=on
  charging (Preq is neg) : RelationalOperator  Operator=<  RndMeth=Nearest  InputSameDT=on
  "discharge max power allowed (-0.1 is for safety, to prevent taking the square of a tiny -ive # in I=I(P) elsewhere)" : Fcn  Expr=(u[1]-u[2])*u[2]/u[3]-0.1
  ess minimum voltage : Constant  Value=ess_min_volts
  ess_module_num : Gain  Gain=ess_module_num  SaturateOnIntegerOverflow=on  OutDataTypeStr=Inherit: Same as input  ParamDataTypeStr=Inherit: Same as input
  limit by battery max or min mc voltage or ess min : MinMax  Function=max  Inputs=3  InputSameDT=on  SaturateOnIntegerOverflow=on
  mc minimum voltage : Constant  Value=mc_min_volts
  min : MinMax  Inputs=2  InputSameDT=on  SaturateOnIntegerOverflow=on
  no power req if SOC<0 and trying  to discharge : Switch  Threshold=eps
  no power req if SOC>.999 and trying  to charge : Switch  Threshold=eps
  "Pbty, limited" : Outport  InitialOutput=0
  wires:
  Constant1/1 -> Relational Operator/2
  Relational Operator/1 -> Logical Operator/1
  Pbty/1 -> Relational Operator3/1, min/1, charging (Preq is neg)/1
  Constant2/1 -> Relational Operator3/2
  Relational Operator3/1 -> Logical Operator/2
  Constant3/1 -> no power req if SOC<0 and trying  to discharge/3
  Logical Operator/1 -> no power req if SOC<0 and trying  to discharge/2, Limits/2(not SOC  low limited)
  Voc/1 -> Mux/1, Gain/1
  min/1 -> no power req if SOC<0 and trying  to discharge/1, Limits/3(power req)
  Mux/1 -> "discharge max power allowed (-0.1 is for safety, to prevent taking the square of a tiny -ive # in I=I(P) elsewhere)"/1
  limit by battery max or min mc voltage or ess min/1 -> Mux/2, Limits/5(V used)
  "discharge max power allowed (-0.1 is for safety, to prevent taking the square of a tiny -ive # in I=I(P) elsewhere)"/1 -> Limits/4(power bat limited), min/2
  mc minimum voltage/1 -> limit by battery max or min mc voltage or ess min/2, Limits/6(V mc_min_volts)
  Rint/1 -> Mux/3
  Gain/1 -> limit by battery max or min mc voltage or ess min/1, Limits/7(V battery (.5Voc))
  ess minimum voltage/1 -> ess_module_num/1
  ess_module_num/1 -> limit by battery max or min mc voltage or ess min/3, Limits/8(V ess_min_volts)
  SOC/1 -> Relational Operator/1, SOC>=.999/1
  SOC>=.999/1 -> Logical Operator1/1
  Constant6/1 -> charging (Preq is neg)/2
  charging (Preq is neg)/1 -> Logical Operator1/2
  Constant5/1 -> SOC>=.999/2
  Constant4/1 -> no power req if SOC>.999 and trying  to charge/1
  no power req if SOC<0 and trying  to discharge/1 -> no power req if SOC>.999 and trying  to charge/3
  no power req if SOC>.999 and trying  to charge/1 -> "Pbty, limited"/1
  Logical Operator1/1 -> no power req if SOC>.999 and trying  to charge/2, Limits/1(SOC  high limited)

== system BD_PAR_AUTO_base_model/energy storage <ess>/ess config/energy storage <ess>/max pack pwr (W)1 ==
  SOC : Inport
  ess_mod_tmp : Inport  Port=2
  #bty : Constant  Value=ess_module_num
  Constant : Constant  Value=mc_min_volts
  Constant1 : Constant  Value=0.001
  Constant2 : Constant  Value=0
  Constant7 : Constant  Value=ess_on
  Gain : Gain  Gain=0.5  SaturateOnIntegerOverflow=on  OutDataTypeStr=Inherit: Same as input  ParamDataTypeStr=Inherit: Same as input
  MinMax1 : MinMax  Function=max  Inputs=3  InputSameDT=on  SaturateOnIntegerOverflow=on
  Mux : Mux  Inputs=3
  Mux3 : Mux  Inputs=3
  Mux5 : Mux  Inputs=3
  Product : Product  InputSameDT=on  RndMeth=Zero  SaturateOnIntegerOverflow=on  OutDataTypeStr=Inherit: Same as first input
  Product3 : Product  InputSameDT=on  RndMeth=Zero  SaturateOnIntegerOverflow=on  OutDataTypeStr=Inherit: Same as first input
  Rchg (ohms)1 : Subsystem  mask(2-D Table Lookup){xindex=ess_tmp, yindex=ess_soc, table=ess_r_chg}
      mask prompts: xindex "X Index"; yindex "Y Index"
      mask help:
      | Two Dimensional Table Lookup
      | The first input corresponds to X Index and the second input corresponds to the Y Index
      mask init:
      | sftab2chk(xindex,yindex,table);
      mask Help: This block returns a linearly interpolated intersection from the table using the X index (which corresponds to the rows of the table) and the Y index (which corresponds to the columns of the table).  Extrapolation is used.
      mask Display: plot(-10,-10,110,110,[90,50,10],[90,40,30],[90,50,10],[50,26,20],[90,50,10],[22,13,10])
  Rdis (ohms) : Subsystem  mask(2-D Table Lookup){xindex=ess_tmp, yindex=ess_soc, table=ess_r_dis}
      mask prompts: xindex "X Index"; yindex "Y Index"
      mask help:
      | Two Dimensional Table Lookup
      | The first input corresponds to X Index and the second input corresponds to the Y Index
      mask init:
      | sftab2chk(xindex,yindex,table);
      mask Help: This block returns a linearly interpolated intersection from the table using the X index (which corresponds to the rows of the table) and the Y index (which corresponds to the columns of the table).  Extrapolation is used.
      mask Display: plot(-10,-10,110,110,[90,50,10],[90,40,30],[90,50,10],[50,26,20],[90,50,10],[22,13,10])
  Relational Operator : RelationalOperator  Operator=>  RndMeth=Nearest  InputSameDT=on
  Switch : Switch  Threshold=eps
  VOC (V) : Subsystem  mask(2-D Table Lookup){xindex=ess_tmp, yindex=ess_soc, table=ess_voc}
      mask prompts: xindex "X Index"; yindex "Y Index"
      mask help:
      | Two Dimensional Table Lookup
      | The first input corresponds to X Index and the second input corresponds to the Y Index
      mask init:
      | sftab2chk(xindex,yindex,table);
      mask Help: This block returns a linearly interpolated intersection from the table using the X index (which corresponds to the rows of the table) and the Y index (which corresponds to the columns of the table).  Extrapolation is used.
      mask Display: plot(-10,-10,110,110,[90,50,10],[90,40,30],[90,50,10],[50,26,20],[90,50,10],[22,13,10])
  Voc-I*R : Fcn  Expr=u[2]-u[1]*u[3]
  and : Logic
  iabs min=(Voc-Vmax)/R : Fcn  Expr=(u(1)-u(2))/u(3)
  max power corresponding to minimum voltage : Fcn  Expr=(u[1]-u[2])*u[2]/u[3]
  min ess V : Constant  Value=ess_module_num*ess_min_volts
  min ess V1 : Constant  Value=ess_module_num*ess_max_volts
  resistance scale fun : Gain  Gain=ess_res_scale_fun(ess_res_scale_coef,ess_module_num,ess_cap_scale)  SaturateOnIntegerOverflow=on  OutDataTypeStr=Inherit: Same as input  ParamDataTypeStr=Inherit: Same as input
  resistance scale fun1 : Gain  Gain=ess_res_scale_fun(ess_res_scale_coef,ess_module_num,ess_cap_scale)  SaturateOnIntegerOverflow=on  OutDataTypeStr=Inherit: Same as input  ParamDataTypeStr=Inherit: Same as input
  max ess discharge pwr : Outport  InitialOutput=0
  max ess charge pwr : Outport  Port=2  InitialOutput=0
  wires:
  #bty/1 -> Product/2
  Rchg (ohms)1/1(table out) -> resistance scale fun/1
  resistance scale fun/1 -> Mux3/3, Mux5/3
  Product3/1 -> max ess charge pwr/1
  Voc-I*R/1 -> Product3/2
  iabs min=(Voc-Vmax)/R/1 -> Product3/1, Mux3/1
  Mux3/1 -> Voc-I*R/1
  Mux5/1 -> iabs min=(Voc-Vmax)/R/1
  min ess V1/1 -> Mux5/2
  Switch/1 -> max ess discharge pwr/1
  SOC/1 -> Rchg (ohms)1/2(y0), Rdis (ohms)/2(y0), VOC (V)/2(y0), Relational Operator/1
  Constant2/1 -> Switch/3
  max power corresponding to minimum voltage/1 -> Switch/1
  Rdis (ohms)/1(table out) -> resistance scale fun1/1
  VOC (V)/1(table out) -> Product/1
  resistance scale fun1/1 -> Mux/3
  Product/1 -> Mux3/2, Mux5/1, Gain/1, Mux/1
  MinMax1/1 -> Mux/2
  Gain/1 -> MinMax1/1
  Mux/1 -> max power corresponding to minimum voltage/1
  Constant/1 -> MinMax1/2
  Constant1/1 -> Relational Operator/2
  ess_mod_tmp/1 -> Rchg (ohms)1/1(x0), Rdis (ohms)/1(x0), VOC (V)/1(x0)
  min ess V/1 -> MinMax1/3
  and/1 -> Switch/2
  Relational Operator/1 -> and/1
  Constant7/1 -> and/2
